simulink model "odefangcheng"  (R2021b)
settings: Solver=VariableStepAuto  StartTime=0.0  StopTime=10.0  RelTol=1e-3
settings Model: Creator=86195  LastModifiedBy=86195

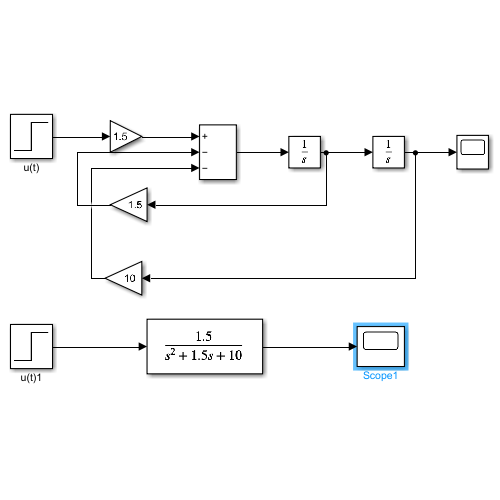
[thumbnail: Simulink's stored preview of the top-level diagram]
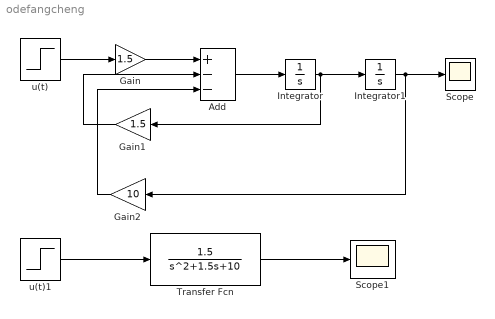
== system odefangcheng ==
  Add : Sum  Inputs=+--
  Gain : Gain  Gain=1.5
  Gain1 : Gain  Gain=1.5
  Gain2 : Gain  Gain=10
  Integrator : Integrator
  Integrator1 : Integrator
  Scope : Scope
  Scope1 : Scope
  Transfer Fcn : TransferFcn  Numerator=[1.5]  Denominator=[1 1.5 10]
  u(t) : Step  Time=0  SampleTime=0
  u(t)1 : Step  Time=0  SampleTime=0
  wires:
  u(t)/1 -> Gain/1
  Gain/1 -> Add/1
  Add/1 -> Integrator/1
  Integrator/1 -> Integrator1/1, Gain1/1
  Integrator1/1 -> Scope/1, Gain2/1
  Gain1/1 -> Add/2
  Gain2/1 -> Add/3
  u(t)1/1 -> Transfer Fcn/1
  Transfer Fcn/1 -> Scope1/1
